simulink model "hclab7test"  (Simulink 7.6)
settings: Solver=ode45  StartTime=0.0  StopTime=10.0  RelTol=1e-3
settings Model: Creator=student  LastModifiedBy=student

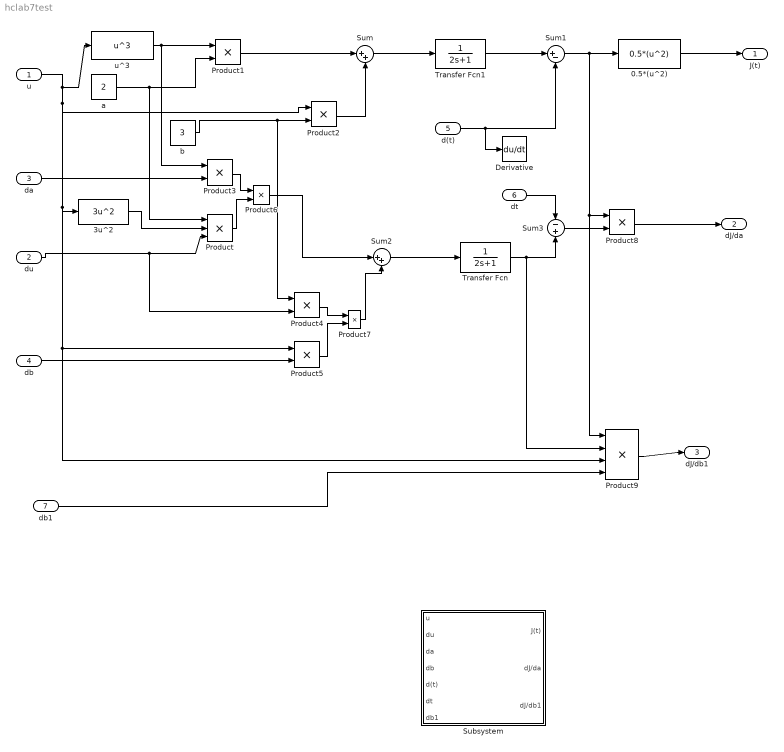
== system hclab7test ==
  u : Inport
  du : Inport  Port=2
  da : Inport  Port=3
  db : Inport  Port=4
  d(t) : Inport  Port=5
  dt : Inport  Port=6
  db1 : Inport  Port=7
  0.5*(u^2) : MATLABFcn  MATLABFcn=0.5*(u^2)
  3u^2 : MATLABFcn  MATLABFcn=3u^2
  Derivative : Derivative
  Product : Product  Inputs=3  RndMeth=Zero
  Product{1..8} (8 alike) : Product  RndMeth=Zero
  Product9 : Product  Inputs=4  RndMeth=Zero
  Subsystem : Subsystem
  Sum : Sum  Inputs=|++
  Sum1 : Sum  Inputs=|+-
  Sum2 : Sum  Inputs=|++
  Sum3 : Sum  Inputs=-|+
  Transfer Fcn : TransferFcn  Denominator=[2 1]
  Transfer Fcn1 : TransferFcn  Denominator=[2 1]
  a : Constant  Value=2
  b : Constant  Value=3
  u^3 : MATLABFcn  MATLABFcn=u^3
  J(t) : Outport
  dJ/da : Outport  Port=2
  dJ/db1 : Outport  Port=3
  wires:
  u/1 -> u^3/1, Product2/1, 3u^2/1, Product5/1, Product9/3
  b/1 -> Product2/2, Product4/1
  u^3/1 -> Product1/1, Product3/1
  a/1 -> Product1/2, Product/1
  3u^2/1 -> Product/2
  du/1 -> Product/3, Product4/2
  Product1/1 -> Sum/1
  da/1 -> Product3/2
  Product6/1 -> Sum2/1
  db/1 -> Product5/2
  Product3/1 -> Product6/1
  Product/1 -> Product6/2
  Product4/1 -> Product7/1
  Product5/1 -> Product7/2
  Product7/1 -> Sum2/2
  Sum2/1 -> Transfer Fcn/1
  Product2/1 -> Sum/2
  Sum/1 -> Transfer Fcn1/1
  Transfer Fcn1/1 -> Sum1/1
  Transfer Fcn/1 -> Sum3/2, Product9/2
  d(t)/1 -> Sum1/2, Derivative/1
  dt/1 -> Sum3/1
  Sum1/1 -> 0.5*(u^2)/1, Product8/1, Product9/1
  Sum3/1 -> Product8/2
  Product8/1 -> dJ/da/1
  0.5*(u^2)/1 -> J(t)/1
  db1/1 -> Product9/4
  Product9/1 -> dJ/db1/1

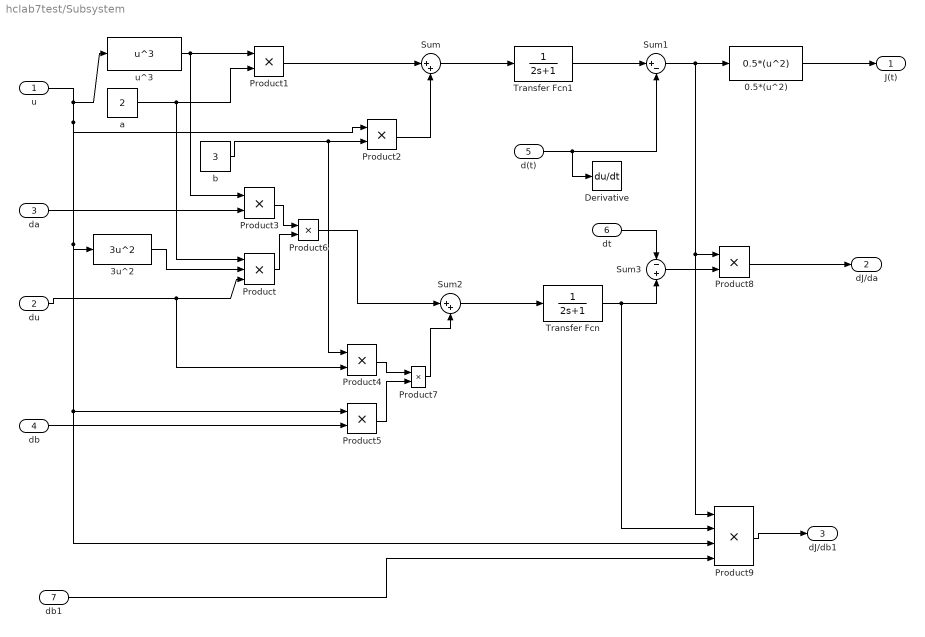
== system hclab7test/Subsystem ==
  u : Inport
  du : Inport  Port=2
  da : Inport  Port=3
  db : Inport  Port=4
  d(t) : Inport  Port=5
  dt : Inport  Port=6
  db1 : Inport  Port=7
  0.5*(u^2) : MATLABFcn  MATLABFcn=0.5*(u^2)
  3u^2 : MATLABFcn  MATLABFcn=3u^2
  Derivative : Derivative
  Product : Product  Inputs=3  RndMeth=Zero
  Product{1..8} (8 alike) : Product  RndMeth=Zero
  Product9 : Product  Inputs=4  RndMeth=Zero
  Sum : Sum  Inputs=|++
  Sum1 : Sum  Inputs=|+-
  Sum2 : Sum  Inputs=|++
  Sum3 : Sum  Inputs=-|+
  Transfer Fcn : TransferFcn  Denominator=[2 1]
  Transfer Fcn1 : TransferFcn  Denominator=[2 1]
  a : Constant  Value=2
  b : Constant  Value=3
  u^3 : MATLABFcn  MATLABFcn=u^3
  J(t) : Outport
  dJ/da : Outport  Port=2
  dJ/db1 : Outport  Port=3
  wires:
  u/1 -> u^3/1, Product2/1, 3u^2/1, Product5/1, Product9/3
  b/1 -> Product2/2, Product4/1
  u^3/1 -> Product1/1, Product3/1
  a/1 -> Product1/2, Product/1
  3u^2/1 -> Product/2
  du/1 -> Product/3, Product4/2
  Product1/1 -> Sum/1
  da/1 -> Product3/2
  Product6/1 -> Sum2/1
  db/1 -> Product5/2
  Product3/1 -> Product6/1
  Product/1 -> Product6/2
  Product4/1 -> Product7/1
  Product5/1 -> Product7/2
  Product7/1 -> Sum2/2
  Sum2/1 -> Transfer Fcn/1
  Product2/1 -> Sum/2
  Sum/1 -> Transfer Fcn1/1
  Transfer Fcn1/1 -> Sum1/1
  Transfer Fcn/1 -> Sum3/2, Product9/2
  d(t)/1 -> Sum1/2, Derivative/1
  dt/1 -> Sum3/1
  Sum1/1 -> 0.5*(u^2)/1, Product8/1, Product9/1
  Sum3/1 -> Product8/2
  Product8/1 -> dJ/da/1
  0.5*(u^2)/1 -> J(t)/1
  db1/1 -> Product9/4
  Product9/1 -> dJ/db1/1
